simulink model "Air_Condition"  (R2016b)
settings: Solver=FixedStepDiscrete  StartTime=0.0  StopTime=inf  FixedStep=AirCdn.tiSimnTiStep_C  RelTol=1e-3  EnableMultiTasking=on
settings Model: Creator=djuenema  LastModifiedBy=djuenema
settings DataIOCC: SaveFormat=StructureWithTime  SaveOutput=off  DSMLogging=off  VisualizeSimOutput=off  SaveTime=off  SignalLoggingName=Results
settings OptimizationCC: BlockReduction=off  ConditionallyExecuteInputs=off  LifeSpan=inf
settings DebuggingCC: AllowSymbolicDim=off  SFUnexpectedBacktrackingDiag=warning  SFNoUnconditionalDefaultTransitionDiag=warning  SFExecutionAtInitializationDiag=none
settings ModelReferenceCC: ModelReferenceNumInstancesAllowed=Single  PropagateSignalLabelsOutOfModel=off
settings GRTTargetCC: TargetLangStandard=C89/C90 (ANSI)
settings ConfigComp: CovMetricSettings=dw  CovHtmlReporting=on  CovSaveCumulativeToWorkspaceVar=on  CovSaveSingleToWorkspaceVar=on  CovExternalEMLEnable=off

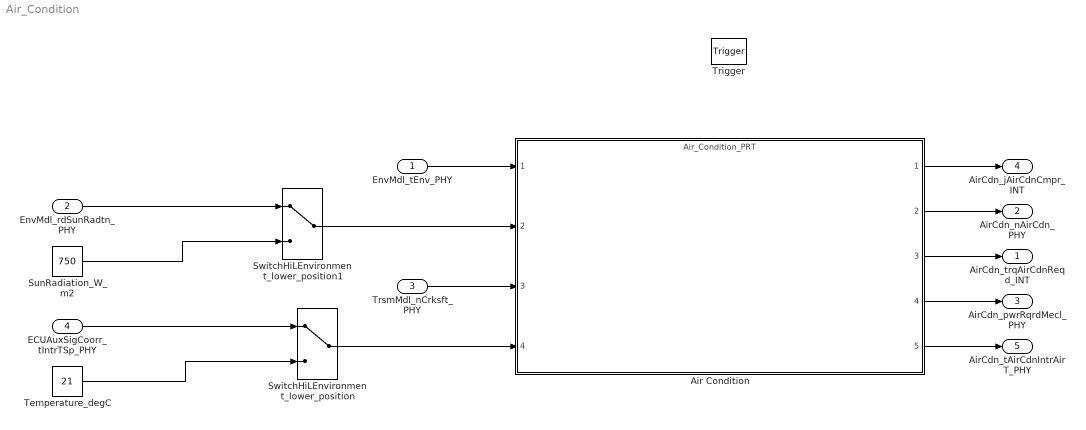
== system Air_Condition ==
  EnvMdl_tEnv_PHY : Inport
  EnvMdl_rdSunRadtn_PHY : Inport  Port=2
  TrsmMdl_nCrksft_PHY : Inport  Port=3
  ECUAuxSigCoorr_tIntrTSp_PHY : Inport  Port=4
  Trigger : TriggerPort  TriggerType=function-call  VariantControl=Variant  PortDimensions=1
  Air Condition : ModelReference  ModelNameDialog=Air_Condition_PRT.slxp  ModelReferenceVersion=1.3  CopyOfModelProtected=on
  SunRadiation_W_m2 : Constant  Value=750
  SwitchHiLEnvironment_lower_position : ManualSwitch
  SwitchHiLEnvironment_lower_position1 : ManualSwitch
  Temperature_degC : Constant  Value=21
  AirCdn_trqAirCdnReqd_INT : Outport
  AirCdn_nAirCdn_PHY : Outport  Port=2
  AirCdn_pwrRqrdMecl_PHY : Outport  Port=3
  AirCdn_jAirCdnCmpr_INT : Outport  Port=4
  AirCdn_tAirCdnIntrAirT_PHY : Outport  Port=5
  wires:
  TrsmMdl_nCrksft_PHY/1 -> Air Condition/3
  EnvMdl_tEnv_PHY/1 -> Air Condition/1
  EnvMdl_rdSunRadtn_PHY/1 -> SwitchHiLEnvironment_lower_position1/1
  Air Condition/4 -> AirCdn_pwrRqrdMecl_PHY/1
  Air Condition/3 -> AirCdn_trqAirCdnReqd_INT/1
  Air Condition/2 -> AirCdn_nAirCdn_PHY/1
  Air Condition/1 -> AirCdn_jAirCdnCmpr_INT/1
  Temperature_degC/1 -> SwitchHiLEnvironment_lower_position/2
  Air Condition/5 -> AirCdn_tAirCdnIntrAirT_PHY/1
  SunRadiation_W_m2/1 -> SwitchHiLEnvironment_lower_position1/2
  ECUAuxSigCoorr_tIntrTSp_PHY/1 -> SwitchHiLEnvironment_lower_position/1
  SwitchHiLEnvironment_lower_position/1 -> Air Condition/4
  SwitchHiLEnvironment_lower_position1/1 -> Air Condition/2
